simulink model "c7mdde3"  (Simulink 7.7)
settings: Solver=ode45  StartTime=0.0  StopTime=10.0  RelTol=1e-7
PreLoadFcn:
  | A2=diag([0.02,0.03,0.04]);
  | A1=[-13,3,-3; 106,-116,62; 207,-207,113]; B=[0; 1; 2];
settings Model: Creator=Professor Dingyu Xue  LastModifiedBy=Professor Dingyu Xue
settings DataIOCC: SignalLoggingName=sigsOut
settings DebuggingCC: SaveWithParameterizedLinksMsg=none  SignalResolutionControl=TryResolveAllWithWarning  SolverPrmCheckMsg=none  MultiTaskDSMMsg=warning  MultiTaskCondExecSysMsg=none  StrictBusMsg=None
settings HardwareCC: TargetUnknown=on
settings RTWCC: IncludeERTFirstTime=on

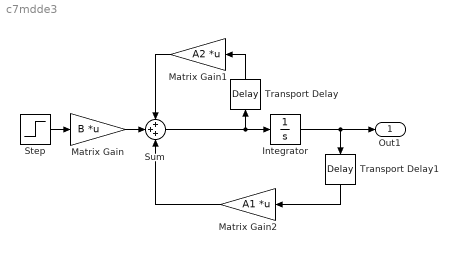
== system c7mdde3 ==
  Integrator : Integrator
  Matrix Gain : Gain  Gain=B  Multiplication=Matrix(K*u)  SaturateOnIntegerOverflow=on  OutDataTypeStr=Inherit: Same as input  ParamDataTypeStr=Inherit: Same as input
  Matrix Gain1 : Gain  Gain=A2  Multiplication=Matrix(K*u)  SaturateOnIntegerOverflow=on  OutDataTypeStr=Inherit: Same as input  ParamDataTypeStr=Inherit: Same as input
  Matrix Gain2 : Gain  Gain=A1  Multiplication=Matrix(K*u)  SaturateOnIntegerOverflow=on  OutDataTypeStr=Inherit: Same as input  ParamDataTypeStr=Inherit: Same as input
  Step : Step  Time=0  SampleTime=0
  Sum : Sum  Inputs=+++  SaturateOnIntegerOverflow=on
  Transport Delay : TransportDelay  DelayTime=0.5
  Transport Delay1 : TransportDelay  DelayTime=0.15
  Out1 : Outport
  wires:
  Sum/1 -> Integrator/1, Transport Delay/1
  Transport Delay/1 -> Matrix Gain1/1
  Matrix Gain1/1 -> Sum/1
  Integrator/1 -> Transport Delay1/1, Out1/1
  Transport Delay1/1 -> Matrix Gain2/1
  Matrix Gain2/1 -> Sum/3
  Matrix Gain/1 -> Sum/2
  Step/1 -> Matrix Gain/1
